simulink model "bergeron_100_segments"  (R2025b)
settings: Solver=FixedStepAuto  StartTime=0.0  StopTime=5/60  RelTol=1e-3
undefined symbols (not defined in the file): C0, C1, L0, L1, R0, R1, Ts
libraries: ee_lib_for_power_systems x200, ee_lib x5, nesl_utility x2, fl_lib x1
settings Model: Creator=gdudgeon  LastModifiedBy=gdudgeon

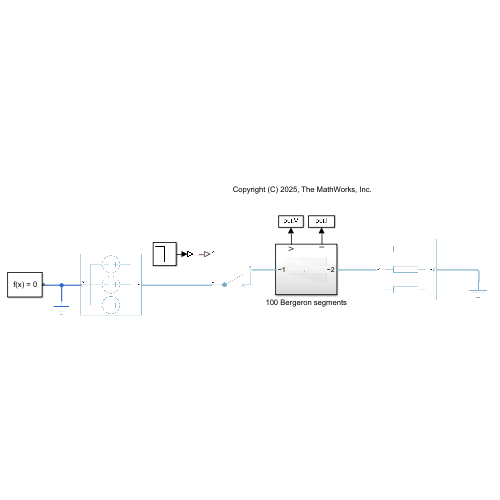
[thumbnail: Simulink's stored preview of the top-level diagram]
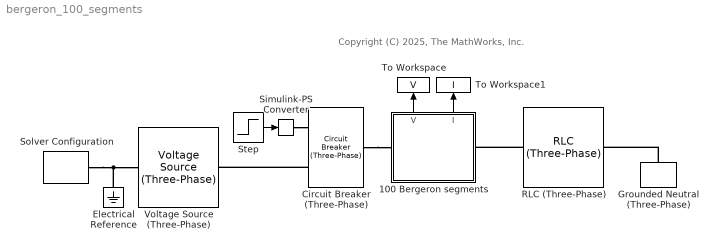
== system bergeron_100_segments ==
  note: Copyright (C) 2025, The MathWorks, Inc.
  100 Bergeron segments : Subsystem
      settings: PortSchema="{\"entries\":[{\"content\":{\"sides\":[{\"content\":{\"connectorIds\":[\"LConn1\"]},\"type\":\"ConnectorPlacement.EquallySpacedRectSide\",\"uuid\":\"b99b41a7-961a-494a-ac92-0b0e7e7066d5\"},{\"content\":{\"connectorIds\":[\"RConn1\"],\"side\":\"RIGHT\"},\"type\":\"ConnectorPlacement.EquallySpacedRectSide\",\"uuid\":\"a32a1a94-e4d8-4756-b184-838770a8045e\"},{\"content\":{\"connectorIds\":[\"Out1\",\"Out2\"],\"side\":\"TOP\"},\"type\":\"ConnectorPlacement.EquallySpacedRectSide\",\"uuid\":\"26c359be-d192-4d53-9097-18fe14f1011c\"},{\"content\":{\"side\":\"BOTTOM\"},\"type\":\"ConnectorPlacement.EquallySpacedRectSide\",\"uuid\":\"027abb80-d680-4e4d-9999-4a3aa56ae95f\"}]},\"type\":\"ConnectorPlacement.EquallySpacedConnector\",\"uuid\":\"03c9bddf-ebbb-4b3d-af53-face1d9ef075\"}],\"packageUris\":[\"http://schema.mathworks.com/mf0/Connector/R2020b\"],\"version\":\"1.0\"}"
  Circuit Breaker (Three-Phase) : ee_lib/Switches & Breakers/Circuit Breaker (Three-Phase)  R_closed=1e-6 Ohm  G_open=1e-6 1/Ohm  threshold=0.5 V  breaker_behavior=ee.enum.switches.breakerBehavior.zeroCrossingEnable
      settings: InternalSimscapePortConfiguration="{\"Bottom\":[],\"Left\":[{\"id\":\"vT\",\"label\":\"vT\",\"type\":\"input\"},{\"id\":\"N1\",\"label\":\"~1\",\"type\":\"foundation.electrical.three_phase\"}],\"Right\":[{\"id\":\"N2\",\"label\":\"~2\",\"type\":\"foundation.electrical.three_phase\"}],\"Top\":[]}"
  Electrical Reference : fl_lib/Electrical/Electrical Elements/Electrical Reference
  Grounded Neutral (Three-Phase) : ee_lib/Connectors & References/Grounded Neutral (Three-Phase)
  RLC (Three-Phase) : ee_lib/Passive/RLC Assemblies/RLC (Three-Phase)  port_option=ee.enum.threePhasePort.composite  component_structure=ee.enum.rlc.structure.SeriesRL  R=100 Ohm  L=1e-3 H  C=1e-6 F  R_parasitic=0 Ohm  G_parasitic=0 1/Ohm  IL_specify=off  IL_priority=High  IL=[0, 0, 0] A  IL_nominal_specify=off  IL_nominal_value=1  IL_nominal_unit=A  VC_specify=off  VC_priority=High  VC=[0, 0, 0] V  VC_nominal_specify=off  VC_nominal_value=1  VC_nominal_unit=V
      settings: InternalSimscapePortConfiguration="{\"Bottom\":[],\"Left\":[{\"id\":\"N1\",\"label\":\"~1\",\"type\":\"foundation.electrical.three_phase\"}],\"Right\":[{\"id\":\"N2\",\"label\":\"~2\",\"type\":\"foundation.electrical.three_phase\"}],\"Top\":[]}"
  Simulink-PS Converter : nesl_utility/Simulink-PS Converter  PhysicalDomain=network_engine_domain  SubClassName=ps_input  LeftPortType=input  RightPortType=output  PseudoPeriodic=off  Frequencies=[]  NoiseDistribution=none  NoiseParameters=[]  Unit=1  AffineConversion=off  FilteringAndDerivatives=provide  SimscapeFilterOrder=1  InputFilterTimeConstant=0.001  UdotUserProvided=0
  Solver Configuration : nesl_utility/Solver Configuration  PhysicalDomain=network_engine_domain  SubClassName=solver  LeftPortType=input  RightPortType=generic  Tones=[]  Harmonics=[]  SimulateNoise=off  Profile=off  UseLocalSampling=off  EnableSwitchedLinearOptims=on  FrequencyDomain=off  UseCCode=off  RelTol=0.001  AbsTol=0.001  MinStep=1e-09  ToWorkspace=off  RevertToSquareIcSolve=off  NumHomotopyIterations=100  PhasorMode=off  PhasorModeNumHarmonics=1  ConsistencySolver=NEWTON_XTOL_AFTER_FTOL  IndexReductionMethod=None  DoDC=off  ResidualTolerance=1e-09  ConsistencyTolSource=GLOBAL  ConsistencyAbsTol=0.001  ConsistencyRelTol=0.001  ConsistencyTolFactor=0.001  UseLocalSolver=on  LocalSolverChoice=NE_PARTITIONING_ADVANCER  ResolveIndetEquations=off  FunctionEvalNumThread=1  LocalSolverSampleTime=Ts  DoFixedCost=off  MaxNonlinIter=1  MaxModeIter=2  ComputeImpulses=off  ImpulseIterations=2  LinearAlgebra=auto  LinearAlgebraNumThread=0  EquationFormulation=NE_TIME_EF  DelaysMemoryBudget=1024  AutomaticFiltering=off  FilteringTimeConstant=0.001  PartitionStorageMethod=AS_NEEDED  PartitionMemoryBudget=1024  PartitionMethod=ROBUST  MultibodyUseLocalSolver=off  MultibodyLocalSolverChoice=ODE1  MultibodyLocalSolverSampleTime=0.001
  Step : Step  Time=0.1/60  Before=1  After=0  SampleTime=0
  To Workspace : ToWorkspace  VariableName=V  SaveFormat=Timeseries  SampleTime=Ts
  To Workspace1 : ToWorkspace  VariableName=I  SaveFormat=Timeseries  SampleTime=Ts
  Voltage Source (Three-Phase) : ee_lib/Sources/Voltage Source (Three-Phase)  vline_rms=100 V  shift=0 deg  freq=60 Hz  impedance_option=4  SShortCircuit=1e6 A*V  XR=15  R=0.01 Ohm  L=3.97e-4 H  harmonic_option=0  harmonic_orders=[5, 7, 11, 13]  harmonic_ratios=[.1, .1, .1, .1]  G_parasitic=0 1/Ohm  I_specify=off  I_priority=None  I=[0, 0, 0] A  I_nominal_specify=off  I_nominal_value=1  I_nominal_unit=A
  wires:
  Step/1 -> Simulink-PS Converter/1
  100 Bergeron segments/2(I) -> To Workspace1/1
  100 Bergeron segments/1(V) -> To Workspace/1
  connections:
  Electrical Reference/LConn1 -- Voltage Source (Three-Phase)/LConn1 -- Solver Configuration/RConn1
  Grounded Neutral (Three-Phase)/LConn1 -- RLC (Three-Phase)/RConn1
  Circuit Breaker (Three-Phase)/LConn2 -- Voltage Source (Three-Phase)/RConn1
  Circuit Breaker (Three-Phase)/RConn1 -- 100 Bergeron segments/LConn1
  RLC (Three-Phase)/LConn1 -- 100 Bergeron segments/RConn1
  Simulink-PS Converter/RConn1 -- Circuit Breaker (Three-Phase)/LConn1

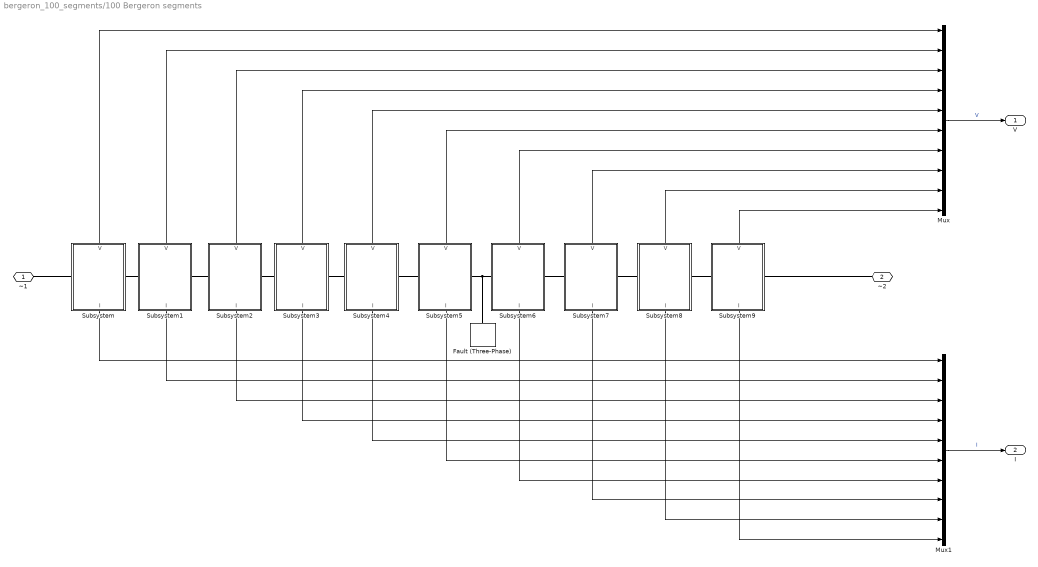
== system bergeron_100_segments/100 Bergeron segments ==
  Fault (Three-Phase) : ee_lib/Utilities/Fault (Three-Phase)  fault_type_option=11  R_pn_fault=1e-3 Ohm  R_ng_fault=1e-3 Ohm  exposemeasurement=ee.enum.exposemeasurement.hidden  enable_external_fault=ee.enum.external_fault.hidden  fault_threshold=0.5  fault_condition=1  fault_resettable=0  enable_temporal_fault=1  fault_start_time=2/60 s  fault_duration=0.001 s  G_parasitic=1e-6 1/Ohm
      settings: InternalSimscapePortConfiguration="{\"Bottom\":[],\"Left\":[{\"id\":\"N\",\"label\":\"~\",\"type\":\"foundation.electrical.three_phase\"}],\"Right\":[],\"Top\":[]}"
  Mux : Mux  Inputs=10
  Mux1 : Mux  Inputs=10
  Subsystem : Subsystem
      settings: PortSchema="{\"entries\":[{\"content\":{\"sides\":[{\"content\":{\"connectorIds\":[\"LConn1\"]},\"type\":\"ConnectorPlacement.EquallySpacedRectSide\",\"uuid\":\"be24dfa2-f72c-4790-92c4-42d34f360bf9\"},{\"content\":{\"connectorIds\":[\"RConn1\"],\"side\":\"RIGHT\"},\"type\":\"ConnectorPlacement.EquallySpacedRectSide\",\"uuid\":\"712463f8-85c9-4ba1-8bf5-09eaf7a29451\"},{\"content\":{\"connectorIds\":[\"Out2\"],\"side\":\"TOP\"},\"type\":\"ConnectorPlacement.EquallySpacedRectSide\",\"uuid\":\"03bd5c26-7b85-49ce-a0e2-a017bb2912ae\"},{\"content\":{\"connectorIds\":[\"Out1\"],\"side\":\"BOTTOM\"},\"type\":\"ConnectorPlacement.EquallySpacedRectSide\",\"uuid\":\"03e5b7e0-a176-4f73-96e3-dc5cabc5b21e\"}]},\"type\":\"ConnectorPlacement.EquallySpacedConnector\",\"uuid\":\"4458ec78-2ee4-4806-a1a7-ced2cc432a6e\"}],\"packageUris\":[\"http://schema.mathworks.com/mf0/Connector/R2020b\"],\"version\":\"1.0\"}"
  Subsystem1 : Subsystem
      settings: PortSchema="{\"entries\":[{\"content\":{\"sides\":[{\"content\":{\"connectorIds\":[\"LConn1\"]},\"type\":\"ConnectorPlacement.EquallySpacedRectSide\",\"uuid\":\"be24dfa2-f72c-4790-92c4-42d34f360bf9\"},{\"content\":{\"connectorIds\":[\"RConn1\"],\"side\":\"RIGHT\"},\"type\":\"ConnectorPlacement.EquallySpacedRectSide\",\"uuid\":\"712463f8-85c9-4ba1-8bf5-09eaf7a29451\"},{\"content\":{\"connectorIds\":[\"Out2\"],\"side\":\"TOP\"},\"type\":\"ConnectorPlacement.EquallySpacedRectSide\",\"uuid\":\"03bd5c26-7b85-49ce-a0e2-a017bb2912ae\"},{\"content\":{\"connectorIds\":[\"Out1\"],\"side\":\"BOTTOM\"},\"type\":\"ConnectorPlacement.EquallySpacedRectSide\",\"uuid\":\"03e5b7e0-a176-4f73-96e3-dc5cabc5b21e\"}]},\"type\":\"ConnectorPlacement.EquallySpacedConnector\",\"uuid\":\"4458ec78-2ee4-4806-a1a7-ced2cc432a6e\"}],\"packageUris\":[\"http://schema.mathworks.com/mf0/Connector/R2020b\"],\"version\":\"1.0\"}"
  Subsystem2 : Subsystem
      settings: PortSchema="{\"entries\":[{\"content\":{\"sides\":[{\"content\":{\"connectorIds\":[\"LConn1\"]},\"type\":\"ConnectorPlacement.EquallySpacedRectSide\",\"uuid\":\"be24dfa2-f72c-4790-92c4-42d34f360bf9\"},{\"content\":{\"connectorIds\":[\"RConn1\"],\"side\":\"RIGHT\"},\"type\":\"ConnectorPlacement.EquallySpacedRectSide\",\"uuid\":\"712463f8-85c9-4ba1-8bf5-09eaf7a29451\"},{\"content\":{\"connectorIds\":[\"Out2\"],\"side\":\"TOP\"},\"type\":\"ConnectorPlacement.EquallySpacedRectSide\",\"uuid\":\"03bd5c26-7b85-49ce-a0e2-a017bb2912ae\"},{\"content\":{\"connectorIds\":[\"Out1\"],\"side\":\"BOTTOM\"},\"type\":\"ConnectorPlacement.EquallySpacedRectSide\",\"uuid\":\"03e5b7e0-a176-4f73-96e3-dc5cabc5b21e\"}]},\"type\":\"ConnectorPlacement.EquallySpacedConnector\",\"uuid\":\"4458ec78-2ee4-4806-a1a7-ced2cc432a6e\"}],\"packageUris\":[\"http://schema.mathworks.com/mf0/Connector/R2020b\"],\"version\":\"1.0\"}"
  Subsystem3 : Subsystem
      settings: PortSchema="{\"entries\":[{\"content\":{\"sides\":[{\"content\":{\"connectorIds\":[\"LConn1\"]},\"type\":\"ConnectorPlacement.EquallySpacedRectSide\",\"uuid\":\"be24dfa2-f72c-4790-92c4-42d34f360bf9\"},{\"content\":{\"connectorIds\":[\"RConn1\"],\"side\":\"RIGHT\"},\"type\":\"ConnectorPlacement.EquallySpacedRectSide\",\"uuid\":\"712463f8-85c9-4ba1-8bf5-09eaf7a29451\"},{\"content\":{\"connectorIds\":[\"Out2\"],\"side\":\"TOP\"},\"type\":\"ConnectorPlacement.EquallySpacedRectSide\",\"uuid\":\"03bd5c26-7b85-49ce-a0e2-a017bb2912ae\"},{\"content\":{\"connectorIds\":[\"Out1\"],\"side\":\"BOTTOM\"},\"type\":\"ConnectorPlacement.EquallySpacedRectSide\",\"uuid\":\"03e5b7e0-a176-4f73-96e3-dc5cabc5b21e\"}]},\"type\":\"ConnectorPlacement.EquallySpacedConnector\",\"uuid\":\"4458ec78-2ee4-4806-a1a7-ced2cc432a6e\"}],\"packageUris\":[\"http://schema.mathworks.com/mf0/Connector/R2020b\"],\"version\":\"1.0\"}"
  Subsystem4 : Subsystem
      settings: PortSchema="{\"entries\":[{\"content\":{\"sides\":[{\"content\":{\"connectorIds\":[\"LConn1\"]},\"type\":\"ConnectorPlacement.EquallySpacedRectSide\",\"uuid\":\"be24dfa2-f72c-4790-92c4-42d34f360bf9\"},{\"content\":{\"connectorIds\":[\"RConn1\"],\"side\":\"RIGHT\"},\"type\":\"ConnectorPlacement.EquallySpacedRectSide\",\"uuid\":\"712463f8-85c9-4ba1-8bf5-09eaf7a29451\"},{\"content\":{\"connectorIds\":[\"Out2\"],\"side\":\"TOP\"},\"type\":\"ConnectorPlacement.EquallySpacedRectSide\",\"uuid\":\"03bd5c26-7b85-49ce-a0e2-a017bb2912ae\"},{\"content\":{\"connectorIds\":[\"Out1\"],\"side\":\"BOTTOM\"},\"type\":\"ConnectorPlacement.EquallySpacedRectSide\",\"uuid\":\"03e5b7e0-a176-4f73-96e3-dc5cabc5b21e\"}]},\"type\":\"ConnectorPlacement.EquallySpacedConnector\",\"uuid\":\"4458ec78-2ee4-4806-a1a7-ced2cc432a6e\"}],\"packageUris\":[\"http://schema.mathworks.com/mf0/Connector/R2020b\"],\"version\":\"1.0\"}"
  Subsystem5 : Subsystem
      settings: PortSchema="{\"entries\":[{\"content\":{\"sides\":[{\"content\":{\"connectorIds\":[\"LConn1\"]},\"type\":\"ConnectorPlacement.EquallySpacedRectSide\",\"uuid\":\"be24dfa2-f72c-4790-92c4-42d34f360bf9\"},{\"content\":{\"connectorIds\":[\"RConn1\"],\"side\":\"RIGHT\"},\"type\":\"ConnectorPlacement.EquallySpacedRectSide\",\"uuid\":\"712463f8-85c9-4ba1-8bf5-09eaf7a29451\"},{\"content\":{\"connectorIds\":[\"Out2\"],\"side\":\"TOP\"},\"type\":\"ConnectorPlacement.EquallySpacedRectSide\",\"uuid\":\"03bd5c26-7b85-49ce-a0e2-a017bb2912ae\"},{\"content\":{\"connectorIds\":[\"Out1\"],\"side\":\"BOTTOM\"},\"type\":\"ConnectorPlacement.EquallySpacedRectSide\",\"uuid\":\"03e5b7e0-a176-4f73-96e3-dc5cabc5b21e\"}]},\"type\":\"ConnectorPlacement.EquallySpacedConnector\",\"uuid\":\"4458ec78-2ee4-4806-a1a7-ced2cc432a6e\"}],\"packageUris\":[\"http://schema.mathworks.com/mf0/Connector/R2020b\"],\"version\":\"1.0\"}"
  Subsystem6 : Subsystem
      settings: PortSchema="{\"entries\":[{\"content\":{\"sides\":[{\"content\":{\"connectorIds\":[\"LConn1\"]},\"type\":\"ConnectorPlacement.EquallySpacedRectSide\",\"uuid\":\"be24dfa2-f72c-4790-92c4-42d34f360bf9\"},{\"content\":{\"connectorIds\":[\"RConn1\"],\"side\":\"RIGHT\"},\"type\":\"ConnectorPlacement.EquallySpacedRectSide\",\"uuid\":\"712463f8-85c9-4ba1-8bf5-09eaf7a29451\"},{\"content\":{\"connectorIds\":[\"Out2\"],\"side\":\"TOP\"},\"type\":\"ConnectorPlacement.EquallySpacedRectSide\",\"uuid\":\"03bd5c26-7b85-49ce-a0e2-a017bb2912ae\"},{\"content\":{\"connectorIds\":[\"Out1\"],\"side\":\"BOTTOM\"},\"type\":\"ConnectorPlacement.EquallySpacedRectSide\",\"uuid\":\"03e5b7e0-a176-4f73-96e3-dc5cabc5b21e\"}]},\"type\":\"ConnectorPlacement.EquallySpacedConnector\",\"uuid\":\"4458ec78-2ee4-4806-a1a7-ced2cc432a6e\"}],\"packageUris\":[\"http://schema.mathworks.com/mf0/Connector/R2020b\"],\"version\":\"1.0\"}"
  Subsystem7 : Subsystem
      settings: PortSchema="{\"entries\":[{\"content\":{\"sides\":[{\"content\":{\"connectorIds\":[\"LConn1\"]},\"type\":\"ConnectorPlacement.EquallySpacedRectSide\",\"uuid\":\"be24dfa2-f72c-4790-92c4-42d34f360bf9\"},{\"content\":{\"connectorIds\":[\"RConn1\"],\"side\":\"RIGHT\"},\"type\":\"ConnectorPlacement.EquallySpacedRectSide\",\"uuid\":\"712463f8-85c9-4ba1-8bf5-09eaf7a29451\"},{\"content\":{\"connectorIds\":[\"Out2\"],\"side\":\"TOP\"},\"type\":\"ConnectorPlacement.EquallySpacedRectSide\",\"uuid\":\"03bd5c26-7b85-49ce-a0e2-a017bb2912ae\"},{\"content\":{\"connectorIds\":[\"Out1\"],\"side\":\"BOTTOM\"},\"type\":\"ConnectorPlacement.EquallySpacedRectSide\",\"uuid\":\"03e5b7e0-a176-4f73-96e3-dc5cabc5b21e\"}]},\"type\":\"ConnectorPlacement.EquallySpacedConnector\",\"uuid\":\"4458ec78-2ee4-4806-a1a7-ced2cc432a6e\"}],\"packageUris\":[\"http://schema.mathworks.com/mf0/Connector/R2020b\"],\"version\":\"1.0\"}"
  Subsystem8 : Subsystem
      settings: PortSchema="{\"entries\":[{\"content\":{\"sides\":[{\"content\":{\"connectorIds\":[\"LConn1\"]},\"type\":\"ConnectorPlacement.EquallySpacedRectSide\",\"uuid\":\"be24dfa2-f72c-4790-92c4-42d34f360bf9\"},{\"content\":{\"connectorIds\":[\"RConn1\"],\"side\":\"RIGHT\"},\"type\":\"ConnectorPlacement.EquallySpacedRectSide\",\"uuid\":\"712463f8-85c9-4ba1-8bf5-09eaf7a29451\"},{\"content\":{\"connectorIds\":[\"Out2\"],\"side\":\"TOP\"},\"type\":\"ConnectorPlacement.EquallySpacedRectSide\",\"uuid\":\"03bd5c26-7b85-49ce-a0e2-a017bb2912ae\"},{\"content\":{\"connectorIds\":[\"Out1\"],\"side\":\"BOTTOM\"},\"type\":\"ConnectorPlacement.EquallySpacedRectSide\",\"uuid\":\"03e5b7e0-a176-4f73-96e3-dc5cabc5b21e\"}]},\"type\":\"ConnectorPlacement.EquallySpacedConnector\",\"uuid\":\"4458ec78-2ee4-4806-a1a7-ced2cc432a6e\"}],\"packageUris\":[\"http://schema.mathworks.com/mf0/Connector/R2020b\"],\"version\":\"1.0\"}"
  Subsystem9 : Subsystem
      settings: PortSchema="{\"entries\":[{\"content\":{\"sides\":[{\"content\":{\"connectorIds\":[\"LConn1\"]},\"type\":\"ConnectorPlacement.EquallySpacedRectSide\",\"uuid\":\"be24dfa2-f72c-4790-92c4-42d34f360bf9\"},{\"content\":{\"connectorIds\":[\"RConn1\"],\"side\":\"RIGHT\"},\"type\":\"ConnectorPlacement.EquallySpacedRectSide\",\"uuid\":\"712463f8-85c9-4ba1-8bf5-09eaf7a29451\"},{\"content\":{\"connectorIds\":[\"Out2\"],\"side\":\"TOP\"},\"type\":\"ConnectorPlacement.EquallySpacedRectSide\",\"uuid\":\"03bd5c26-7b85-49ce-a0e2-a017bb2912ae\"},{\"content\":{\"connectorIds\":[\"Out1\"],\"side\":\"BOTTOM\"},\"type\":\"ConnectorPlacement.EquallySpacedRectSide\",\"uuid\":\"03e5b7e0-a176-4f73-96e3-dc5cabc5b21e\"}]},\"type\":\"ConnectorPlacement.EquallySpacedConnector\",\"uuid\":\"4458ec78-2ee4-4806-a1a7-ced2cc432a6e\"}],\"packageUris\":[\"http://schema.mathworks.com/mf0/Connector/R2020b\"],\"version\":\"1.0\"}"
  ~1 : PMIOPort  Side=Left
  ~2 : PMIOPort  Port=2  Side=Right
  V : Outport
  I : Outport  Port=2
  wires:
  Subsystem9/1(I) -> Mux1/10
  Subsystem2/2(V) -> Mux/3
  Subsystem2/1(I) -> Mux1/3
  Subsystem1/2(V) -> Mux/2
  Subsystem6/2(V) -> Mux/7
  Subsystem5/1(I) -> Mux1/6
  Subsystem4/2(V) -> Mux/5
  Subsystem7/1(I) -> Mux1/8
  Subsystem7/2(V) -> Mux/8
  Subsystem5/2(V) -> Mux/6
  Subsystem/1(I) -> Mux1/1
  Subsystem6/1(I) -> Mux1/7
  Subsystem8/2(V) -> Mux/9
  Subsystem9/2(V) -> Mux/10
  Subsystem8/1(I) -> Mux1/9
  Subsystem3/1(I) -> Mux1/4
  Subsystem3/2(V) -> Mux/4
  Subsystem/2(V) -> Mux/1
  Subsystem4/1(I) -> Mux1/5
  Subsystem1/1(I) -> Mux1/2
  Mux1/1 -> I/1  "I"
  Mux/1 -> V/1  "V"
  connections:
  Subsystem3/RConn1 -- Subsystem4/LConn1
  Subsystem/LConn1 -- ~1/RConn1
  Subsystem9/RConn1 -- ~2/RConn1
  Subsystem7/LConn1 -- Subsystem6/RConn1
  Subsystem8/LConn1 -- Subsystem7/RConn1
  Fault (Three-Phase)/LConn1 -- Subsystem5/RConn1 -- Subsystem6/LConn1
  Subsystem5/LConn1 -- Subsystem4/RConn1
  Subsystem1/LConn1 -- Subsystem/RConn1
  Subsystem3/LConn1 -- Subsystem2/RConn1
  Subsystem2/LConn1 -- Subsystem1/RConn1
  Subsystem9/LConn1 -- Subsystem8/RConn1

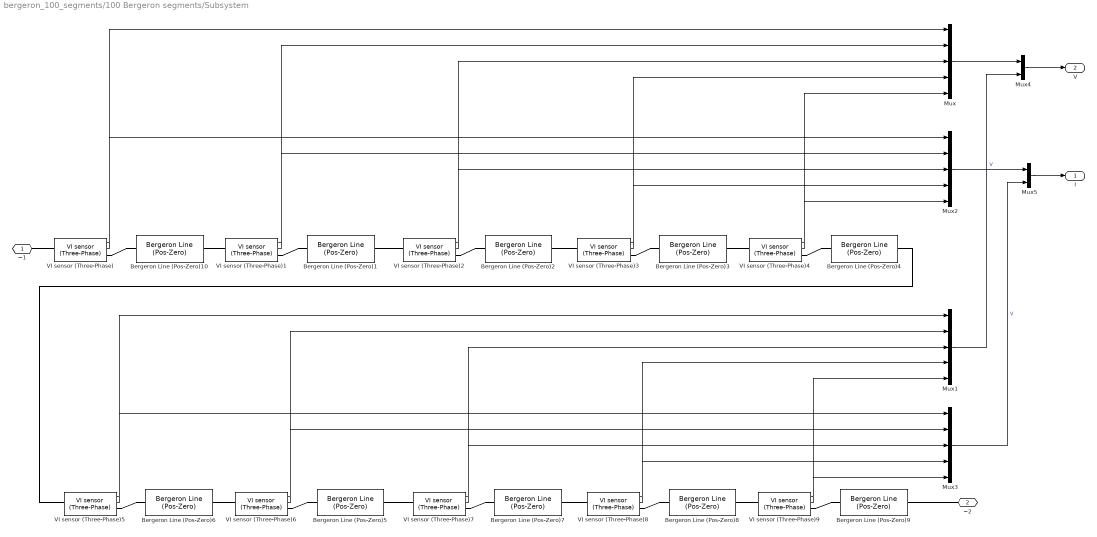
== system bergeron_100_segments/100 Bergeron segments/Subsystem ==
  Bergeron Line (Pos-Zero){1..10} (10 alike) : ee_lib_for_power_systems/Network Components/Bergeron Line (Pos-Zero)  length=length  R1_L1_C1=[R1 L1 C1]  R0_L0_C0=[R0 L0 C0]  Ts=Ts
      settings: SourceProductName=Support Library for Power Systems
  Mux{,1..3} (4 alike) : Mux  Inputs=5
  Mux4 : Mux  Inputs=2
  Mux5 : Mux  Inputs=2
  VI sensor (Three-Phase){,1..9} (10 alike) : ee_lib_for_power_systems/Sense and Measure/VI sensor (Three-Phase)  volt_meas=Phase-to-Ground (Phase Voltage)  meas_units=SI  Vnom=24e3  Pnom=100e6
      settings: SourceProductName=Support Library for Power Systems
  ~1 : PMIOPort  Side=Left
  ~2 : PMIOPort  Port=2  Side=Right
  I : Outport
  V : Outport  Port=2
  wires:
  VI sensor (Three-Phase)/1 -> Mux/1
  VI sensor (Three-Phase)1/1 -> Mux/2
  VI sensor (Three-Phase)2/1 -> Mux/3
  VI sensor (Three-Phase)3/1 -> Mux/4
  VI sensor (Three-Phase)4/1 -> Mux/5
  VI sensor (Three-Phase)/2 -> Mux2/1
  VI sensor (Three-Phase)1/2 -> Mux2/2
  VI sensor (Three-Phase)2/2 -> Mux2/3
  VI sensor (Three-Phase)3/2 -> Mux2/4
  VI sensor (Three-Phase)4/2 -> Mux2/5
  VI sensor (Three-Phase)5/1 -> Mux1/1
  VI sensor (Three-Phase)6/1 -> Mux1/2
  VI sensor (Three-Phase)7/1 -> Mux1/3
  VI sensor (Three-Phase)8/1 -> Mux1/4
  VI sensor (Three-Phase)9/1 -> Mux1/5
  VI sensor (Three-Phase)5/2 -> Mux3/1
  VI sensor (Three-Phase)6/2 -> Mux3/2
  VI sensor (Three-Phase)7/2 -> Mux3/3
  VI sensor (Three-Phase)8/2 -> Mux3/4
  VI sensor (Three-Phase)9/2 -> Mux3/5
  Mux/1 -> Mux4/1
  Mux1/1 -> Mux4/2
  Mux4/1 -> V/1
  Mux2/1 -> Mux5/1  "V"
  Mux3/1 -> Mux5/2  "V"
  Mux5/1 -> I/1
  connections:
  Bergeron Line (Pos-Zero)10/LConn1 -- VI sensor (Three-Phase)/RConn1
  VI sensor (Three-Phase)/LConn1 -- ~1/RConn1
  VI sensor (Three-Phase)1/LConn1 -- Bergeron Line (Pos-Zero)10/RConn1
  ~2/RConn1 -- Bergeron Line (Pos-Zero)9/RConn1
  Bergeron Line (Pos-Zero)1/LConn1 -- VI sensor (Three-Phase)1/RConn1
  Bergeron Line (Pos-Zero)2/LConn1 -- VI sensor (Three-Phase)2/RConn1
  VI sensor (Three-Phase)2/LConn1 -- Bergeron Line (Pos-Zero)1/RConn1
  Bergeron Line (Pos-Zero)3/LConn1 -- VI sensor (Three-Phase)3/RConn1
  VI sensor (Three-Phase)3/LConn1 -- Bergeron Line (Pos-Zero)2/RConn1
  Bergeron Line (Pos-Zero)4/LConn1 -- VI sensor (Three-Phase)4/RConn1
  Bergeron Line (Pos-Zero)3/RConn1 -- VI sensor (Three-Phase)4/LConn1
  Bergeron Line (Pos-Zero)8/RConn1 -- VI sensor (Three-Phase)9/LConn1
  Bergeron Line (Pos-Zero)9/LConn1 -- VI sensor (Three-Phase)9/RConn1
  VI sensor (Three-Phase)7/LConn1 -- Bergeron Line (Pos-Zero)5/RConn1
  Bergeron Line (Pos-Zero)8/LConn1 -- VI sensor (Three-Phase)8/RConn1
  Bergeron Line (Pos-Zero)7/LConn1 -- VI sensor (Three-Phase)7/RConn1
  Bergeron Line (Pos-Zero)5/LConn1 -- VI sensor (Three-Phase)6/RConn1
  VI sensor (Three-Phase)6/LConn1 -- Bergeron Line (Pos-Zero)6/RConn1
  Bergeron Line (Pos-Zero)6/LConn1 -- VI sensor (Three-Phase)5/RConn1
  VI sensor (Three-Phase)8/LConn1 -- Bergeron Line (Pos-Zero)7/RConn1
  VI sensor (Three-Phase)5/LConn1 -- Bergeron Line (Pos-Zero)4/RConn1

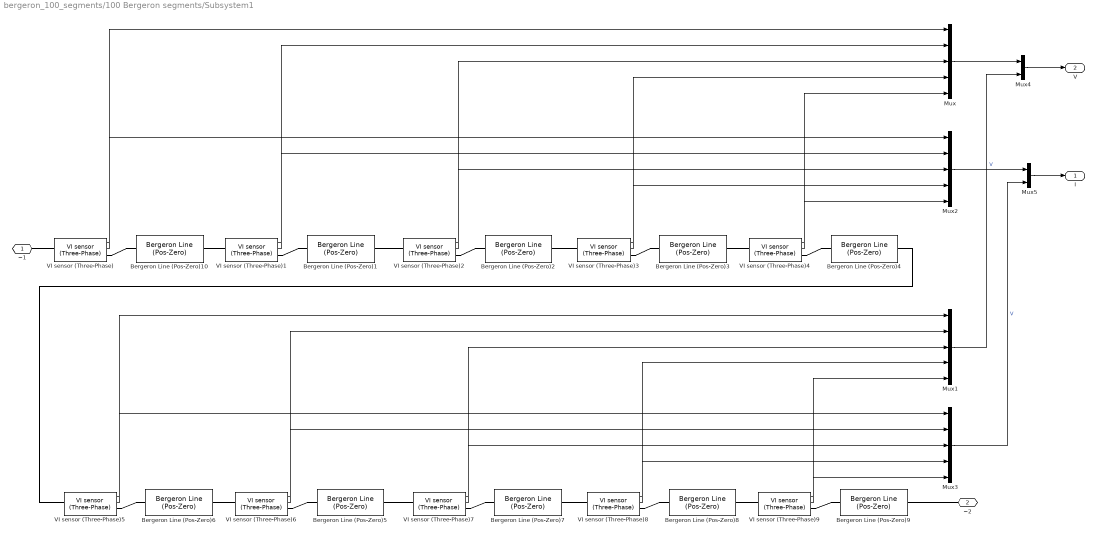
== system bergeron_100_segments/100 Bergeron segments/Subsystem1 ==
  Bergeron Line (Pos-Zero){1..10} (10 alike) : ee_lib_for_power_systems/Network Components/Bergeron Line (Pos-Zero)  length=length  R1_L1_C1=[R1 L1 C1]  R0_L0_C0=[R0 L0 C0]  Ts=Ts
      settings: SourceProductName=Support Library for Power Systems
  Mux{,1..3} (4 alike) : Mux  Inputs=5
  Mux4 : Mux  Inputs=2
  Mux5 : Mux  Inputs=2
  VI sensor (Three-Phase){,1..9} (10 alike) : ee_lib_for_power_systems/Sense and Measure/VI sensor (Three-Phase)  volt_meas=Phase-to-Ground (Phase Voltage)  meas_units=SI  Vnom=24e3  Pnom=100e6
      settings: SourceProductName=Support Library for Power Systems
  ~1 : PMIOPort  Side=Left
  ~2 : PMIOPort  Port=2  Side=Right
  I : Outport
  V : Outport  Port=2
  wires:
  Mux5/1 -> I/1
  Mux3/1 -> Mux5/2  "V"
  Mux2/1 -> Mux5/1  "V"
  Mux4/1 -> V/1
  Mux1/1 -> Mux4/2
  Mux/1 -> Mux4/1
  VI sensor (Three-Phase)9/2 -> Mux3/5
  VI sensor (Three-Phase)8/2 -> Mux3/4
  VI sensor (Three-Phase)7/2 -> Mux3/3
  VI sensor (Three-Phase)6/2 -> Mux3/2
  VI sensor (Three-Phase)5/2 -> Mux3/1
  VI sensor (Three-Phase)9/1 -> Mux1/5
  VI sensor (Three-Phase)8/1 -> Mux1/4
  VI sensor (Three-Phase)7/1 -> Mux1/3
  VI sensor (Three-Phase)6/1 -> Mux1/2
  VI sensor (Three-Phase)5/1 -> Mux1/1
  VI sensor (Three-Phase)4/2 -> Mux2/5
  VI sensor (Three-Phase)3/2 -> Mux2/4
  VI sensor (Three-Phase)2/2 -> Mux2/3
  VI sensor (Three-Phase)1/2 -> Mux2/2
  VI sensor (Three-Phase)/2 -> Mux2/1
  VI sensor (Three-Phase)4/1 -> Mux/5
  VI sensor (Three-Phase)3/1 -> Mux/4
  VI sensor (Three-Phase)2/1 -> Mux/3
  VI sensor (Three-Phase)1/1 -> Mux/2
  VI sensor (Three-Phase)/1 -> Mux/1
  connections:
  VI sensor (Three-Phase)5/LConn1 -- Bergeron Line (Pos-Zero)4/RConn1
  VI sensor (Three-Phase)8/LConn1 -- Bergeron Line (Pos-Zero)7/RConn1
  Bergeron Line (Pos-Zero)6/LConn1 -- VI sensor (Three-Phase)5/RConn1
  VI sensor (Three-Phase)6/LConn1 -- Bergeron Line (Pos-Zero)6/RConn1
  Bergeron Line (Pos-Zero)5/LConn1 -- VI sensor (Three-Phase)6/RConn1
  Bergeron Line (Pos-Zero)7/LConn1 -- VI sensor (Three-Phase)7/RConn1
  Bergeron Line (Pos-Zero)8/LConn1 -- VI sensor (Three-Phase)8/RConn1
  VI sensor (Three-Phase)7/LConn1 -- Bergeron Line (Pos-Zero)5/RConn1
  Bergeron Line (Pos-Zero)9/LConn1 -- VI sensor (Three-Phase)9/RConn1
  Bergeron Line (Pos-Zero)8/RConn1 -- VI sensor (Three-Phase)9/LConn1
  Bergeron Line (Pos-Zero)3/RConn1 -- VI sensor (Three-Phase)4/LConn1
  Bergeron Line (Pos-Zero)4/LConn1 -- VI sensor (Three-Phase)4/RConn1
  VI sensor (Three-Phase)3/LConn1 -- Bergeron Line (Pos-Zero)2/RConn1
  Bergeron Line (Pos-Zero)3/LConn1 -- VI sensor (Three-Phase)3/RConn1
  VI sensor (Three-Phase)2/LConn1 -- Bergeron Line (Pos-Zero)1/RConn1
  Bergeron Line (Pos-Zero)2/LConn1 -- VI sensor (Three-Phase)2/RConn1
  Bergeron Line (Pos-Zero)1/LConn1 -- VI sensor (Three-Phase)1/RConn1
  ~2/RConn1 -- Bergeron Line (Pos-Zero)9/RConn1
  VI sensor (Three-Phase)1/LConn1 -- Bergeron Line (Pos-Zero)10/RConn1
  VI sensor (Three-Phase)/LConn1 -- ~1/RConn1
  Bergeron Line (Pos-Zero)10/LConn1 -- VI sensor (Three-Phase)/RConn1

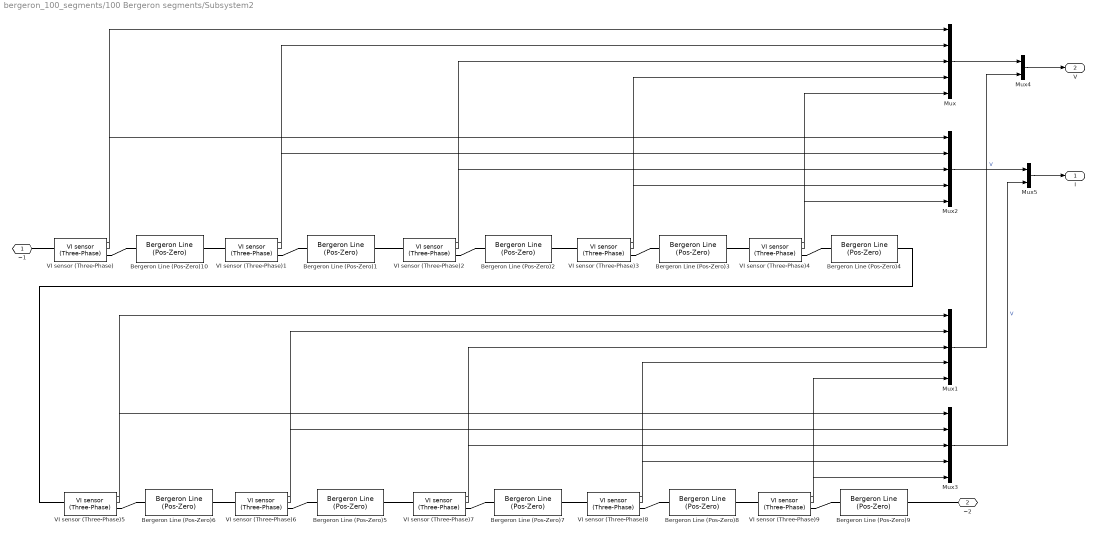
== system bergeron_100_segments/100 Bergeron segments/Subsystem2 ==
  Bergeron Line (Pos-Zero){1..10} (10 alike) : ee_lib_for_power_systems/Network Components/Bergeron Line (Pos-Zero)  length=length  R1_L1_C1=[R1 L1 C1]  R0_L0_C0=[R0 L0 C0]  Ts=Ts
      settings: SourceProductName=Support Library for Power Systems
  Mux{,1..3} (4 alike) : Mux  Inputs=5
  Mux4 : Mux  Inputs=2
  Mux5 : Mux  Inputs=2
  VI sensor (Three-Phase){,1..9} (10 alike) : ee_lib_for_power_systems/Sense and Measure/VI sensor (Three-Phase)  volt_meas=Phase-to-Ground (Phase Voltage)  meas_units=SI  Vnom=24e3  Pnom=100e6
      settings: SourceProductName=Support Library for Power Systems
  ~1 : PMIOPort  Side=Left
  ~2 : PMIOPort  Port=2  Side=Right
  I : Outport
  V : Outport  Port=2
  wires:
  VI sensor (Three-Phase)/1 -> Mux/1
  VI sensor (Three-Phase)1/1 -> Mux/2
  VI sensor (Three-Phase)2/1 -> Mux/3
  VI sensor (Three-Phase)3/1 -> Mux/4
  VI sensor (Three-Phase)4/1 -> Mux/5
  VI sensor (Three-Phase)/2 -> Mux2/1
  VI sensor (Three-Phase)1/2 -> Mux2/2
  VI sensor (Three-Phase)2/2 -> Mux2/3
  VI sensor (Three-Phase)3/2 -> Mux2/4
  VI sensor (Three-Phase)4/2 -> Mux2/5
  VI sensor (Three-Phase)5/1 -> Mux1/1
  VI sensor (Three-Phase)6/1 -> Mux1/2
  VI sensor (Three-Phase)7/1 -> Mux1/3
  VI sensor (Three-Phase)8/1 -> Mux1/4
  VI sensor (Three-Phase)9/1 -> Mux1/5
  VI sensor (Three-Phase)5/2 -> Mux3/1
  VI sensor (Three-Phase)6/2 -> Mux3/2
  VI sensor (Three-Phase)7/2 -> Mux3/3
  VI sensor (Three-Phase)8/2 -> Mux3/4
  VI sensor (Three-Phase)9/2 -> Mux3/5
  Mux/1 -> Mux4/1
  Mux1/1 -> Mux4/2
  Mux4/1 -> V/1
  Mux2/1 -> Mux5/1  "V"
  Mux3/1 -> Mux5/2  "V"
  Mux5/1 -> I/1
  connections:
  Bergeron Line (Pos-Zero)10/LConn1 -- VI sensor (Three-Phase)/RConn1
  VI sensor (Three-Phase)/LConn1 -- ~1/RConn1
  VI sensor (Three-Phase)1/LConn1 -- Bergeron Line (Pos-Zero)10/RConn1
  ~2/RConn1 -- Bergeron Line (Pos-Zero)9/RConn1
  Bergeron Line (Pos-Zero)1/LConn1 -- VI sensor (Three-Phase)1/RConn1
  Bergeron Line (Pos-Zero)2/LConn1 -- VI sensor (Three-Phase)2/RConn1
  VI sensor (Three-Phase)2/LConn1 -- Bergeron Line (Pos-Zero)1/RConn1
  Bergeron Line (Pos-Zero)3/LConn1 -- VI sensor (Three-Phase)3/RConn1
  VI sensor (Three-Phase)3/LConn1 -- Bergeron Line (Pos-Zero)2/RConn1
  Bergeron Line (Pos-Zero)4/LConn1 -- VI sensor (Three-Phase)4/RConn1
  Bergeron Line (Pos-Zero)3/RConn1 -- VI sensor (Three-Phase)4/LConn1
  Bergeron Line (Pos-Zero)8/RConn1 -- VI sensor (Three-Phase)9/LConn1
  Bergeron Line (Pos-Zero)9/LConn1 -- VI sensor (Three-Phase)9/RConn1
  VI sensor (Three-Phase)7/LConn1 -- Bergeron Line (Pos-Zero)5/RConn1
  Bergeron Line (Pos-Zero)8/LConn1 -- VI sensor (Three-Phase)8/RConn1
  Bergeron Line (Pos-Zero)7/LConn1 -- VI sensor (Three-Phase)7/RConn1
  Bergeron Line (Pos-Zero)5/LConn1 -- VI sensor (Three-Phase)6/RConn1
  VI sensor (Three-Phase)6/LConn1 -- Bergeron Line (Pos-Zero)6/RConn1
  Bergeron Line (Pos-Zero)6/LConn1 -- VI sensor (Three-Phase)5/RConn1
  VI sensor (Three-Phase)8/LConn1 -- Bergeron Line (Pos-Zero)7/RConn1
  VI sensor (Three-Phase)5/LConn1 -- Bergeron Line (Pos-Zero)4/RConn1

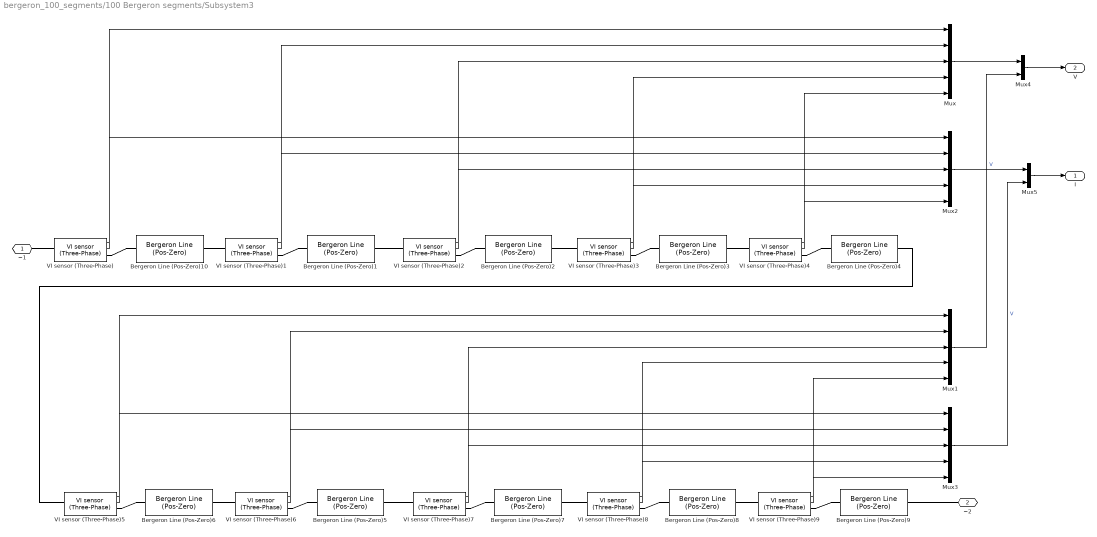
== system bergeron_100_segments/100 Bergeron segments/Subsystem3 ==
  Bergeron Line (Pos-Zero){1..10} (10 alike) : ee_lib_for_power_systems/Network Components/Bergeron Line (Pos-Zero)  length=length  R1_L1_C1=[R1 L1 C1]  R0_L0_C0=[R0 L0 C0]  Ts=Ts
      settings: SourceProductName=Support Library for Power Systems
  Mux{,1..3} (4 alike) : Mux  Inputs=5
  Mux4 : Mux  Inputs=2
  Mux5 : Mux  Inputs=2
  VI sensor (Three-Phase){,1..9} (10 alike) : ee_lib_for_power_systems/Sense and Measure/VI sensor (Three-Phase)  volt_meas=Phase-to-Ground (Phase Voltage)  meas_units=SI  Vnom=24e3  Pnom=100e6
      settings: SourceProductName=Support Library for Power Systems
  ~1 : PMIOPort  Side=Left
  ~2 : PMIOPort  Port=2  Side=Right
  I : Outport
  V : Outport  Port=2
  wires:
  Mux5/1 -> I/1
  Mux3/1 -> Mux5/2  "V"
  Mux2/1 -> Mux5/1  "V"
  Mux4/1 -> V/1
  Mux1/1 -> Mux4/2
  Mux/1 -> Mux4/1
  VI sensor (Three-Phase)9/2 -> Mux3/5
  VI sensor (Three-Phase)8/2 -> Mux3/4
  VI sensor (Three-Phase)7/2 -> Mux3/3
  VI sensor (Three-Phase)6/2 -> Mux3/2
  VI sensor (Three-Phase)5/2 -> Mux3/1
  VI sensor (Three-Phase)9/1 -> Mux1/5
  VI sensor (Three-Phase)8/1 -> Mux1/4
  VI sensor (Three-Phase)7/1 -> Mux1/3
  VI sensor (Three-Phase)6/1 -> Mux1/2
  VI sensor (Three-Phase)5/1 -> Mux1/1
  VI sensor (Three-Phase)4/2 -> Mux2/5
  VI sensor (Three-Phase)3/2 -> Mux2/4
  VI sensor (Three-Phase)2/2 -> Mux2/3
  VI sensor (Three-Phase)1/2 -> Mux2/2
  VI sensor (Three-Phase)/2 -> Mux2/1
  VI sensor (Three-Phase)4/1 -> Mux/5
  VI sensor (Three-Phase)3/1 -> Mux/4
  VI sensor (Three-Phase)2/1 -> Mux/3
  VI sensor (Three-Phase)1/1 -> Mux/2
  VI sensor (Three-Phase)/1 -> Mux/1
  connections:
  VI sensor (Three-Phase)5/LConn1 -- Bergeron Line (Pos-Zero)4/RConn1
  VI sensor (Three-Phase)8/LConn1 -- Bergeron Line (Pos-Zero)7/RConn1
  Bergeron Line (Pos-Zero)6/LConn1 -- VI sensor (Three-Phase)5/RConn1
  VI sensor (Three-Phase)6/LConn1 -- Bergeron Line (Pos-Zero)6/RConn1
  Bergeron Line (Pos-Zero)5/LConn1 -- VI sensor (Three-Phase)6/RConn1
  Bergeron Line (Pos-Zero)7/LConn1 -- VI sensor (Three-Phase)7/RConn1
  Bergeron Line (Pos-Zero)8/LConn1 -- VI sensor (Three-Phase)8/RConn1
  VI sensor (Three-Phase)7/LConn1 -- Bergeron Line (Pos-Zero)5/RConn1
  Bergeron Line (Pos-Zero)9/LConn1 -- VI sensor (Three-Phase)9/RConn1
  Bergeron Line (Pos-Zero)8/RConn1 -- VI sensor (Three-Phase)9/LConn1
  Bergeron Line (Pos-Zero)3/RConn1 -- VI sensor (Three-Phase)4/LConn1
  Bergeron Line (Pos-Zero)4/LConn1 -- VI sensor (Three-Phase)4/RConn1
  VI sensor (Three-Phase)3/LConn1 -- Bergeron Line (Pos-Zero)2/RConn1
  Bergeron Line (Pos-Zero)3/LConn1 -- VI sensor (Three-Phase)3/RConn1
  VI sensor (Three-Phase)2/LConn1 -- Bergeron Line (Pos-Zero)1/RConn1
  Bergeron Line (Pos-Zero)2/LConn1 -- VI sensor (Three-Phase)2/RConn1
  Bergeron Line (Pos-Zero)1/LConn1 -- VI sensor (Three-Phase)1/RConn1
  ~2/RConn1 -- Bergeron Line (Pos-Zero)9/RConn1
  VI sensor (Three-Phase)1/LConn1 -- Bergeron Line (Pos-Zero)10/RConn1
  VI sensor (Three-Phase)/LConn1 -- ~1/RConn1
  Bergeron Line (Pos-Zero)10/LConn1 -- VI sensor (Three-Phase)/RConn1

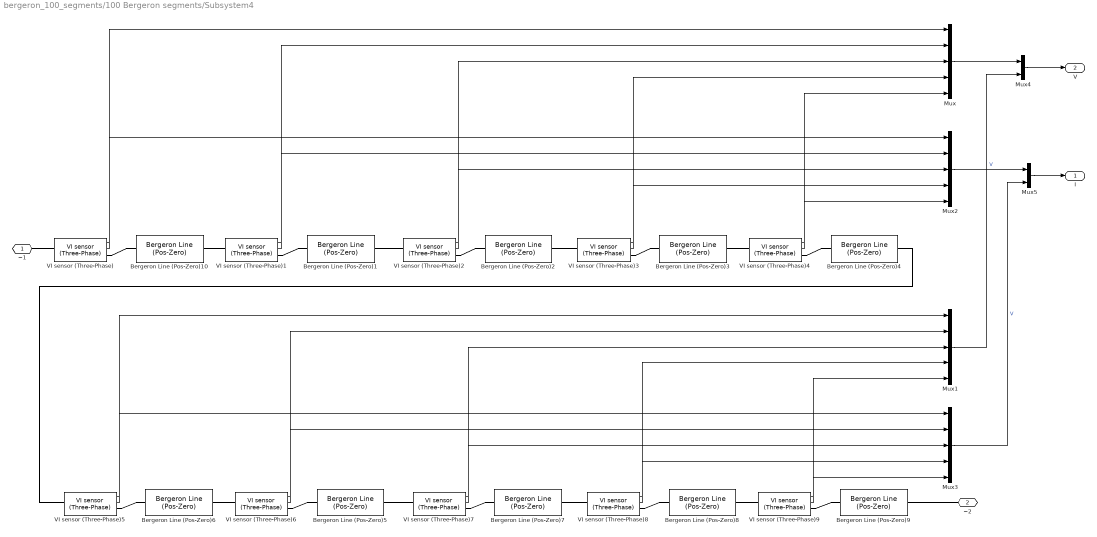
== system bergeron_100_segments/100 Bergeron segments/Subsystem4 ==
  Bergeron Line (Pos-Zero){1..10} (10 alike) : ee_lib_for_power_systems/Network Components/Bergeron Line (Pos-Zero)  length=length  R1_L1_C1=[R1 L1 C1]  R0_L0_C0=[R0 L0 C0]  Ts=Ts
      settings: SourceProductName=Support Library for Power Systems
  Mux{,1..3} (4 alike) : Mux  Inputs=5
  Mux4 : Mux  Inputs=2
  Mux5 : Mux  Inputs=2
  VI sensor (Three-Phase){,1..9} (10 alike) : ee_lib_for_power_systems/Sense and Measure/VI sensor (Three-Phase)  volt_meas=Phase-to-Ground (Phase Voltage)  meas_units=SI  Vnom=24e3  Pnom=100e6
      settings: SourceProductName=Support Library for Power Systems
  ~1 : PMIOPort  Side=Left
  ~2 : PMIOPort  Port=2  Side=Right
  I : Outport
  V : Outport  Port=2
  wires:
  VI sensor (Three-Phase)/1 -> Mux/1
  VI sensor (Three-Phase)1/1 -> Mux/2
  VI sensor (Three-Phase)2/1 -> Mux/3
  VI sensor (Three-Phase)3/1 -> Mux/4
  VI sensor (Three-Phase)4/1 -> Mux/5
  VI sensor (Three-Phase)/2 -> Mux2/1
  VI sensor (Three-Phase)1/2 -> Mux2/2
  VI sensor (Three-Phase)2/2 -> Mux2/3
  VI sensor (Three-Phase)3/2 -> Mux2/4
  VI sensor (Three-Phase)4/2 -> Mux2/5
  VI sensor (Three-Phase)5/1 -> Mux1/1
  VI sensor (Three-Phase)6/1 -> Mux1/2
  VI sensor (Three-Phase)7/1 -> Mux1/3
  VI sensor (Three-Phase)8/1 -> Mux1/4
  VI sensor (Three-Phase)9/1 -> Mux1/5
  VI sensor (Three-Phase)5/2 -> Mux3/1
  VI sensor (Three-Phase)6/2 -> Mux3/2
  VI sensor (Three-Phase)7/2 -> Mux3/3
  VI sensor (Three-Phase)8/2 -> Mux3/4
  VI sensor (Three-Phase)9/2 -> Mux3/5
  Mux/1 -> Mux4/1
  Mux1/1 -> Mux4/2
  Mux4/1 -> V/1
  Mux2/1 -> Mux5/1  "V"
  Mux3/1 -> Mux5/2  "V"
  Mux5/1 -> I/1
  connections:
  Bergeron Line (Pos-Zero)10/LConn1 -- VI sensor (Three-Phase)/RConn1
  VI sensor (Three-Phase)/LConn1 -- ~1/RConn1
  VI sensor (Three-Phase)1/LConn1 -- Bergeron Line (Pos-Zero)10/RConn1
  ~2/RConn1 -- Bergeron Line (Pos-Zero)9/RConn1
  Bergeron Line (Pos-Zero)1/LConn1 -- VI sensor (Three-Phase)1/RConn1
  Bergeron Line (Pos-Zero)2/LConn1 -- VI sensor (Three-Phase)2/RConn1
  VI sensor (Three-Phase)2/LConn1 -- Bergeron Line (Pos-Zero)1/RConn1
  Bergeron Line (Pos-Zero)3/LConn1 -- VI sensor (Three-Phase)3/RConn1
  VI sensor (Three-Phase)3/LConn1 -- Bergeron Line (Pos-Zero)2/RConn1
  Bergeron Line (Pos-Zero)4/LConn1 -- VI sensor (Three-Phase)4/RConn1
  Bergeron Line (Pos-Zero)3/RConn1 -- VI sensor (Three-Phase)4/LConn1
  Bergeron Line (Pos-Zero)8/RConn1 -- VI sensor (Three-Phase)9/LConn1
  Bergeron Line (Pos-Zero)9/LConn1 -- VI sensor (Three-Phase)9/RConn1
  VI sensor (Three-Phase)7/LConn1 -- Bergeron Line (Pos-Zero)5/RConn1
  Bergeron Line (Pos-Zero)8/LConn1 -- VI sensor (Three-Phase)8/RConn1
  Bergeron Line (Pos-Zero)7/LConn1 -- VI sensor (Three-Phase)7/RConn1
  Bergeron Line (Pos-Zero)5/LConn1 -- VI sensor (Three-Phase)6/RConn1
  VI sensor (Three-Phase)6/LConn1 -- Bergeron Line (Pos-Zero)6/RConn1
  Bergeron Line (Pos-Zero)6/LConn1 -- VI sensor (Three-Phase)5/RConn1
  VI sensor (Three-Phase)8/LConn1 -- Bergeron Line (Pos-Zero)7/RConn1
  VI sensor (Three-Phase)5/LConn1 -- Bergeron Line (Pos-Zero)4/RConn1

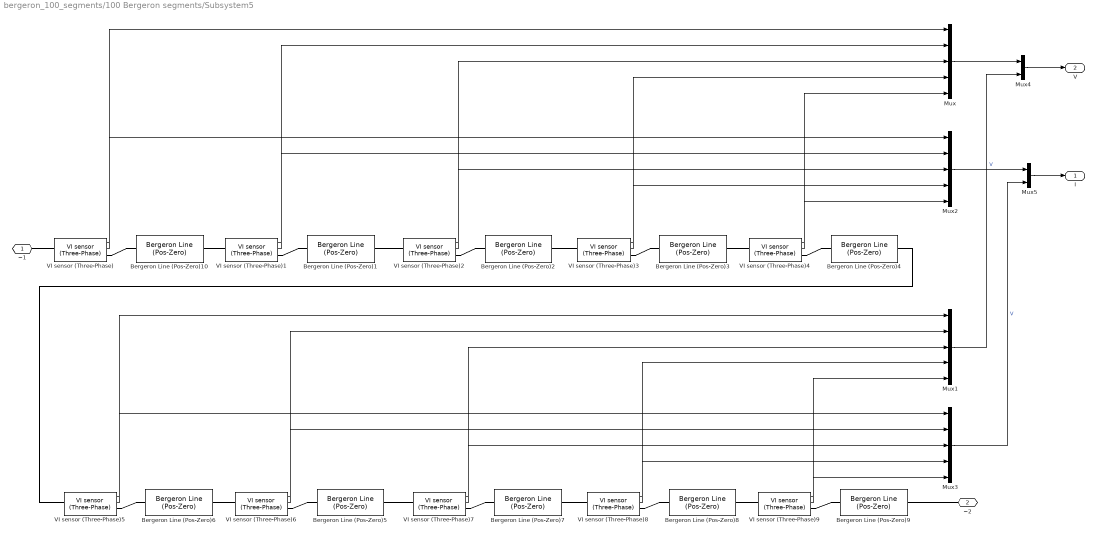
== system bergeron_100_segments/100 Bergeron segments/Subsystem5 ==
  Bergeron Line (Pos-Zero){1..10} (10 alike) : ee_lib_for_power_systems/Network Components/Bergeron Line (Pos-Zero)  length=length  R1_L1_C1=[R1 L1 C1]  R0_L0_C0=[R0 L0 C0]  Ts=Ts
      settings: SourceProductName=Support Library for Power Systems
  Mux{,1..3} (4 alike) : Mux  Inputs=5
  Mux4 : Mux  Inputs=2
  Mux5 : Mux  Inputs=2
  VI sensor (Three-Phase){,1..9} (10 alike) : ee_lib_for_power_systems/Sense and Measure/VI sensor (Three-Phase)  volt_meas=Phase-to-Ground (Phase Voltage)  meas_units=SI  Vnom=24e3  Pnom=100e6
      settings: SourceProductName=Support Library for Power Systems
  ~1 : PMIOPort  Side=Left
  ~2 : PMIOPort  Port=2  Side=Right
  I : Outport
  V : Outport  Port=2
  wires:
  Mux5/1 -> I/1
  Mux3/1 -> Mux5/2  "V"
  Mux2/1 -> Mux5/1  "V"
  Mux4/1 -> V/1
  Mux1/1 -> Mux4/2
  Mux/1 -> Mux4/1
  VI sensor (Three-Phase)9/2 -> Mux3/5
  VI sensor (Three-Phase)8/2 -> Mux3/4
  VI sensor (Three-Phase)7/2 -> Mux3/3
  VI sensor (Three-Phase)6/2 -> Mux3/2
  VI sensor (Three-Phase)5/2 -> Mux3/1
  VI sensor (Three-Phase)9/1 -> Mux1/5
  VI sensor (Three-Phase)8/1 -> Mux1/4
  VI sensor (Three-Phase)7/1 -> Mux1/3
  VI sensor (Three-Phase)6/1 -> Mux1/2
  VI sensor (Three-Phase)5/1 -> Mux1/1
  VI sensor (Three-Phase)4/2 -> Mux2/5
  VI sensor (Three-Phase)3/2 -> Mux2/4
  VI sensor (Three-Phase)2/2 -> Mux2/3
  VI sensor (Three-Phase)1/2 -> Mux2/2
  VI sensor (Three-Phase)/2 -> Mux2/1
  VI sensor (Three-Phase)4/1 -> Mux/5
  VI sensor (Three-Phase)3/1 -> Mux/4
  VI sensor (Three-Phase)2/1 -> Mux/3
  VI sensor (Three-Phase)1/1 -> Mux/2
  VI sensor (Three-Phase)/1 -> Mux/1
  connections:
  VI sensor (Three-Phase)5/LConn1 -- Bergeron Line (Pos-Zero)4/RConn1
  VI sensor (Three-Phase)8/LConn1 -- Bergeron Line (Pos-Zero)7/RConn1
  Bergeron Line (Pos-Zero)6/LConn1 -- VI sensor (Three-Phase)5/RConn1
  VI sensor (Three-Phase)6/LConn1 -- Bergeron Line (Pos-Zero)6/RConn1
  Bergeron Line (Pos-Zero)5/LConn1 -- VI sensor (Three-Phase)6/RConn1
  Bergeron Line (Pos-Zero)7/LConn1 -- VI sensor (Three-Phase)7/RConn1
  Bergeron Line (Pos-Zero)8/LConn1 -- VI sensor (Three-Phase)8/RConn1
  VI sensor (Three-Phase)7/LConn1 -- Bergeron Line (Pos-Zero)5/RConn1
  Bergeron Line (Pos-Zero)9/LConn1 -- VI sensor (Three-Phase)9/RConn1
  Bergeron Line (Pos-Zero)8/RConn1 -- VI sensor (Three-Phase)9/LConn1
  Bergeron Line (Pos-Zero)3/RConn1 -- VI sensor (Three-Phase)4/LConn1
  Bergeron Line (Pos-Zero)4/LConn1 -- VI sensor (Three-Phase)4/RConn1
  VI sensor (Three-Phase)3/LConn1 -- Bergeron Line (Pos-Zero)2/RConn1
  Bergeron Line (Pos-Zero)3/LConn1 -- VI sensor (Three-Phase)3/RConn1
  VI sensor (Three-Phase)2/LConn1 -- Bergeron Line (Pos-Zero)1/RConn1
  Bergeron Line (Pos-Zero)2/LConn1 -- VI sensor (Three-Phase)2/RConn1
  Bergeron Line (Pos-Zero)1/LConn1 -- VI sensor (Three-Phase)1/RConn1
  ~2/RConn1 -- Bergeron Line (Pos-Zero)9/RConn1
  VI sensor (Three-Phase)1/LConn1 -- Bergeron Line (Pos-Zero)10/RConn1
  VI sensor (Three-Phase)/LConn1 -- ~1/RConn1
  Bergeron Line (Pos-Zero)10/LConn1 -- VI sensor (Three-Phase)/RConn1

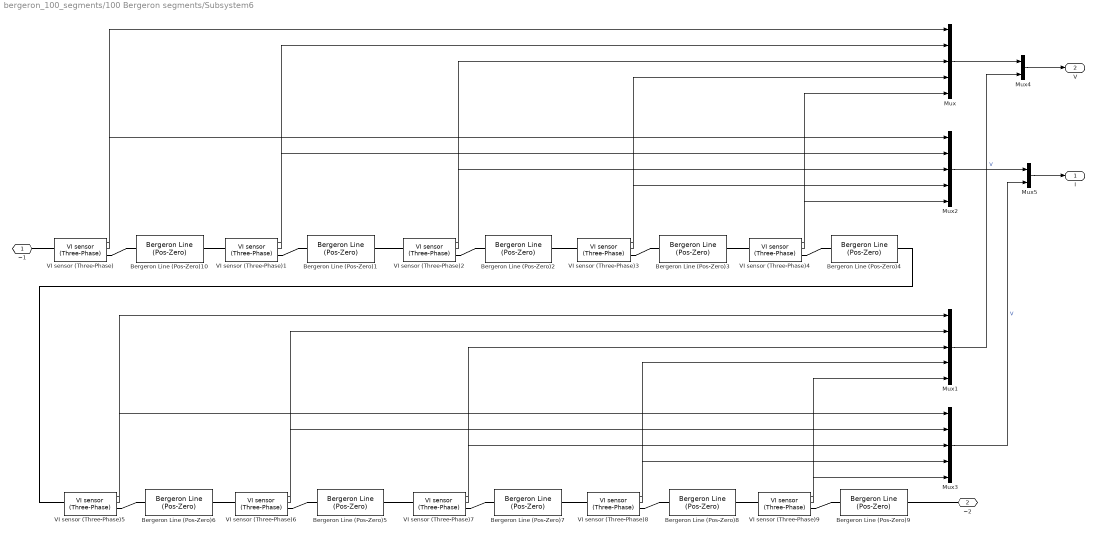
== system bergeron_100_segments/100 Bergeron segments/Subsystem6 ==
  Bergeron Line (Pos-Zero){1..10} (10 alike) : ee_lib_for_power_systems/Network Components/Bergeron Line (Pos-Zero)  length=length  R1_L1_C1=[R1 L1 C1]  R0_L0_C0=[R0 L0 C0]  Ts=Ts
      settings: SourceProductName=Support Library for Power Systems
  Mux{,1..3} (4 alike) : Mux  Inputs=5
  Mux4 : Mux  Inputs=2
  Mux5 : Mux  Inputs=2
  VI sensor (Three-Phase){,1..9} (10 alike) : ee_lib_for_power_systems/Sense and Measure/VI sensor (Three-Phase)  volt_meas=Phase-to-Ground (Phase Voltage)  meas_units=SI  Vnom=24e3  Pnom=100e6
      settings: SourceProductName=Support Library for Power Systems
  ~1 : PMIOPort  Side=Left
  ~2 : PMIOPort  Port=2  Side=Right
  I : Outport
  V : Outport  Port=2
  wires:
  VI sensor (Three-Phase)/1 -> Mux/1
  VI sensor (Three-Phase)1/1 -> Mux/2
  VI sensor (Three-Phase)2/1 -> Mux/3
  VI sensor (Three-Phase)3/1 -> Mux/4
  VI sensor (Three-Phase)4/1 -> Mux/5
  VI sensor (Three-Phase)/2 -> Mux2/1
  VI sensor (Three-Phase)1/2 -> Mux2/2
  VI sensor (Three-Phase)2/2 -> Mux2/3
  VI sensor (Three-Phase)3/2 -> Mux2/4
  VI sensor (Three-Phase)4/2 -> Mux2/5
  VI sensor (Three-Phase)5/1 -> Mux1/1
  VI sensor (Three-Phase)6/1 -> Mux1/2
  VI sensor (Three-Phase)7/1 -> Mux1/3
  VI sensor (Three-Phase)8/1 -> Mux1/4
  VI sensor (Three-Phase)9/1 -> Mux1/5
  VI sensor (Three-Phase)5/2 -> Mux3/1
  VI sensor (Three-Phase)6/2 -> Mux3/2
  VI sensor (Three-Phase)7/2 -> Mux3/3
  VI sensor (Three-Phase)8/2 -> Mux3/4
  VI sensor (Three-Phase)9/2 -> Mux3/5
  Mux/1 -> Mux4/1
  Mux1/1 -> Mux4/2
  Mux4/1 -> V/1
  Mux2/1 -> Mux5/1  "V"
  Mux3/1 -> Mux5/2  "V"
  Mux5/1 -> I/1
  connections:
  Bergeron Line (Pos-Zero)10/LConn1 -- VI sensor (Three-Phase)/RConn1
  VI sensor (Three-Phase)/LConn1 -- ~1/RConn1
  VI sensor (Three-Phase)1/LConn1 -- Bergeron Line (Pos-Zero)10/RConn1
  ~2/RConn1 -- Bergeron Line (Pos-Zero)9/RConn1
  Bergeron Line (Pos-Zero)1/LConn1 -- VI sensor (Three-Phase)1/RConn1
  Bergeron Line (Pos-Zero)2/LConn1 -- VI sensor (Three-Phase)2/RConn1
  VI sensor (Three-Phase)2/LConn1 -- Bergeron Line (Pos-Zero)1/RConn1
  Bergeron Line (Pos-Zero)3/LConn1 -- VI sensor (Three-Phase)3/RConn1
  VI sensor (Three-Phase)3/LConn1 -- Bergeron Line (Pos-Zero)2/RConn1
  Bergeron Line (Pos-Zero)4/LConn1 -- VI sensor (Three-Phase)4/RConn1
  Bergeron Line (Pos-Zero)3/RConn1 -- VI sensor (Three-Phase)4/LConn1
  Bergeron Line (Pos-Zero)8/RConn1 -- VI sensor (Three-Phase)9/LConn1
  Bergeron Line (Pos-Zero)9/LConn1 -- VI sensor (Three-Phase)9/RConn1
  VI sensor (Three-Phase)7/LConn1 -- Bergeron Line (Pos-Zero)5/RConn1
  Bergeron Line (Pos-Zero)8/LConn1 -- VI sensor (Three-Phase)8/RConn1
  Bergeron Line (Pos-Zero)7/LConn1 -- VI sensor (Three-Phase)7/RConn1
  Bergeron Line (Pos-Zero)5/LConn1 -- VI sensor (Three-Phase)6/RConn1
  VI sensor (Three-Phase)6/LConn1 -- Bergeron Line (Pos-Zero)6/RConn1
  Bergeron Line (Pos-Zero)6/LConn1 -- VI sensor (Three-Phase)5/RConn1
  VI sensor (Three-Phase)8/LConn1 -- Bergeron Line (Pos-Zero)7/RConn1
  VI sensor (Three-Phase)5/LConn1 -- Bergeron Line (Pos-Zero)4/RConn1

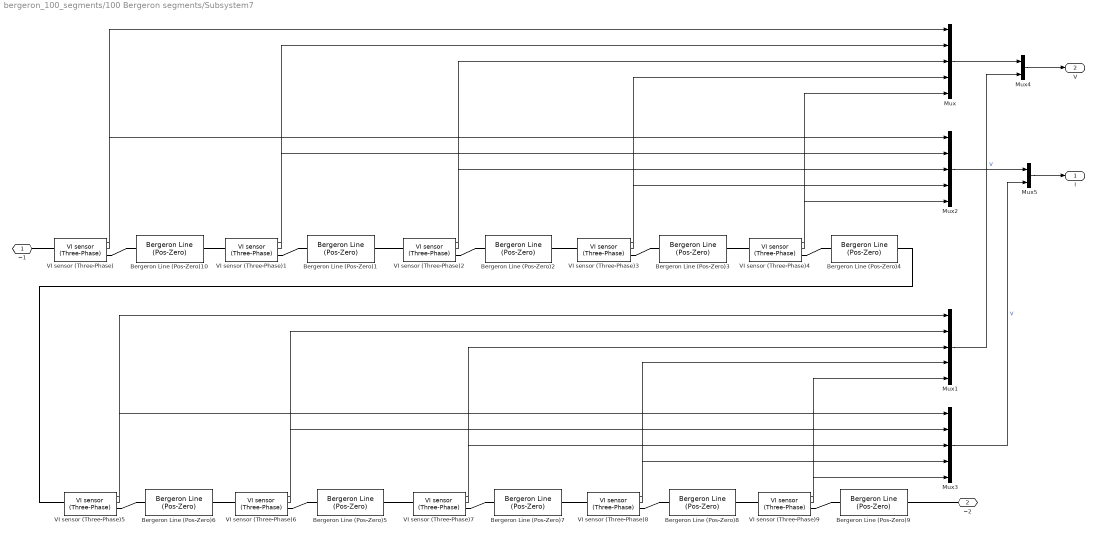
== system bergeron_100_segments/100 Bergeron segments/Subsystem7 ==
  Bergeron Line (Pos-Zero){1..10} (10 alike) : ee_lib_for_power_systems/Network Components/Bergeron Line (Pos-Zero)  length=length  R1_L1_C1=[R1 L1 C1]  R0_L0_C0=[R0 L0 C0]  Ts=Ts
      settings: SourceProductName=Support Library for Power Systems
  Mux{,1..3} (4 alike) : Mux  Inputs=5
  Mux4 : Mux  Inputs=2
  Mux5 : Mux  Inputs=2
  VI sensor (Three-Phase){,1..9} (10 alike) : ee_lib_for_power_systems/Sense and Measure/VI sensor (Three-Phase)  volt_meas=Phase-to-Ground (Phase Voltage)  meas_units=SI  Vnom=24e3  Pnom=100e6
      settings: SourceProductName=Support Library for Power Systems
  ~1 : PMIOPort  Side=Left
  ~2 : PMIOPort  Port=2  Side=Right
  I : Outport
  V : Outport  Port=2
  wires:
  Mux5/1 -> I/1
  Mux3/1 -> Mux5/2  "V"
  Mux2/1 -> Mux5/1  "V"
  Mux4/1 -> V/1
  Mux1/1 -> Mux4/2
  Mux/1 -> Mux4/1
  VI sensor (Three-Phase)9/2 -> Mux3/5
  VI sensor (Three-Phase)8/2 -> Mux3/4
  VI sensor (Three-Phase)7/2 -> Mux3/3
  VI sensor (Three-Phase)6/2 -> Mux3/2
  VI sensor (Three-Phase)5/2 -> Mux3/1
  VI sensor (Three-Phase)9/1 -> Mux1/5
  VI sensor (Three-Phase)8/1 -> Mux1/4
  VI sensor (Three-Phase)7/1 -> Mux1/3
  VI sensor (Three-Phase)6/1 -> Mux1/2
  VI sensor (Three-Phase)5/1 -> Mux1/1
  VI sensor (Three-Phase)4/2 -> Mux2/5
  VI sensor (Three-Phase)3/2 -> Mux2/4
  VI sensor (Three-Phase)2/2 -> Mux2/3
  VI sensor (Three-Phase)1/2 -> Mux2/2
  VI sensor (Three-Phase)/2 -> Mux2/1
  VI sensor (Three-Phase)4/1 -> Mux/5
  VI sensor (Three-Phase)3/1 -> Mux/4
  VI sensor (Three-Phase)2/1 -> Mux/3
  VI sensor (Three-Phase)1/1 -> Mux/2
  VI sensor (Three-Phase)/1 -> Mux/1
  connections:
  VI sensor (Three-Phase)5/LConn1 -- Bergeron Line (Pos-Zero)4/RConn1
  VI sensor (Three-Phase)8/LConn1 -- Bergeron Line (Pos-Zero)7/RConn1
  Bergeron Line (Pos-Zero)6/LConn1 -- VI sensor (Three-Phase)5/RConn1
  VI sensor (Three-Phase)6/LConn1 -- Bergeron Line (Pos-Zero)6/RConn1
  Bergeron Line (Pos-Zero)5/LConn1 -- VI sensor (Three-Phase)6/RConn1
  Bergeron Line (Pos-Zero)7/LConn1 -- VI sensor (Three-Phase)7/RConn1
  Bergeron Line (Pos-Zero)8/LConn1 -- VI sensor (Three-Phase)8/RConn1
  VI sensor (Three-Phase)7/LConn1 -- Bergeron Line (Pos-Zero)5/RConn1
  Bergeron Line (Pos-Zero)9/LConn1 -- VI sensor (Three-Phase)9/RConn1
  Bergeron Line (Pos-Zero)8/RConn1 -- VI sensor (Three-Phase)9/LConn1
  Bergeron Line (Pos-Zero)3/RConn1 -- VI sensor (Three-Phase)4/LConn1
  Bergeron Line (Pos-Zero)4/LConn1 -- VI sensor (Three-Phase)4/RConn1
  VI sensor (Three-Phase)3/LConn1 -- Bergeron Line (Pos-Zero)2/RConn1
  Bergeron Line (Pos-Zero)3/LConn1 -- VI sensor (Three-Phase)3/RConn1
  VI sensor (Three-Phase)2/LConn1 -- Bergeron Line (Pos-Zero)1/RConn1
  Bergeron Line (Pos-Zero)2/LConn1 -- VI sensor (Three-Phase)2/RConn1
  Bergeron Line (Pos-Zero)1/LConn1 -- VI sensor (Three-Phase)1/RConn1
  ~2/RConn1 -- Bergeron Line (Pos-Zero)9/RConn1
  VI sensor (Three-Phase)1/LConn1 -- Bergeron Line (Pos-Zero)10/RConn1
  VI sensor (Three-Phase)/LConn1 -- ~1/RConn1
  Bergeron Line (Pos-Zero)10/LConn1 -- VI sensor (Three-Phase)/RConn1

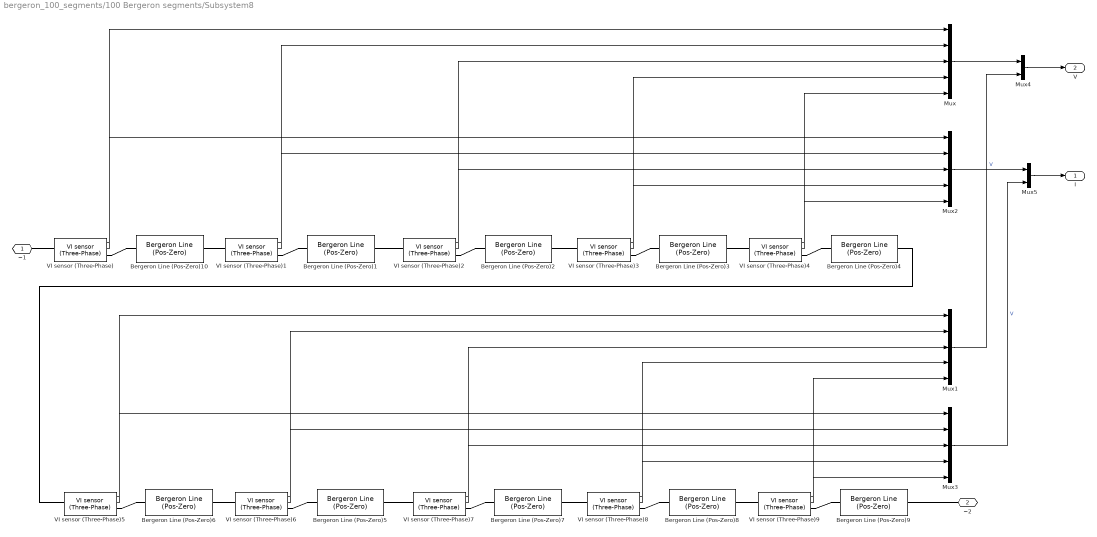
== system bergeron_100_segments/100 Bergeron segments/Subsystem8 ==
  Bergeron Line (Pos-Zero){1..10} (10 alike) : ee_lib_for_power_systems/Network Components/Bergeron Line (Pos-Zero)  length=length  R1_L1_C1=[R1 L1 C1]  R0_L0_C0=[R0 L0 C0]  Ts=Ts
      settings: SourceProductName=Support Library for Power Systems
  Mux{,1..3} (4 alike) : Mux  Inputs=5
  Mux4 : Mux  Inputs=2
  Mux5 : Mux  Inputs=2
  VI sensor (Three-Phase){,1..9} (10 alike) : ee_lib_for_power_systems/Sense and Measure/VI sensor (Three-Phase)  volt_meas=Phase-to-Ground (Phase Voltage)  meas_units=SI  Vnom=24e3  Pnom=100e6
      settings: SourceProductName=Support Library for Power Systems
  ~1 : PMIOPort  Side=Left
  ~2 : PMIOPort  Port=2  Side=Right
  I : Outport
  V : Outport  Port=2
  wires:
  VI sensor (Three-Phase)/1 -> Mux/1
  VI sensor (Three-Phase)1/1 -> Mux/2
  VI sensor (Three-Phase)2/1 -> Mux/3
  VI sensor (Three-Phase)3/1 -> Mux/4
  VI sensor (Three-Phase)4/1 -> Mux/5
  VI sensor (Three-Phase)/2 -> Mux2/1
  VI sensor (Three-Phase)1/2 -> Mux2/2
  VI sensor (Three-Phase)2/2 -> Mux2/3
  VI sensor (Three-Phase)3/2 -> Mux2/4
  VI sensor (Three-Phase)4/2 -> Mux2/5
  VI sensor (Three-Phase)5/1 -> Mux1/1
  VI sensor (Three-Phase)6/1 -> Mux1/2
  VI sensor (Three-Phase)7/1 -> Mux1/3
  VI sensor (Three-Phase)8/1 -> Mux1/4
  VI sensor (Three-Phase)9/1 -> Mux1/5
  VI sensor (Three-Phase)5/2 -> Mux3/1
  VI sensor (Three-Phase)6/2 -> Mux3/2
  VI sensor (Three-Phase)7/2 -> Mux3/3
  VI sensor (Three-Phase)8/2 -> Mux3/4
  VI sensor (Three-Phase)9/2 -> Mux3/5
  Mux/1 -> Mux4/1
  Mux1/1 -> Mux4/2
  Mux4/1 -> V/1
  Mux2/1 -> Mux5/1  "V"
  Mux3/1 -> Mux5/2  "V"
  Mux5/1 -> I/1
  connections:
  Bergeron Line (Pos-Zero)10/LConn1 -- VI sensor (Three-Phase)/RConn1
  VI sensor (Three-Phase)/LConn1 -- ~1/RConn1
  VI sensor (Three-Phase)1/LConn1 -- Bergeron Line (Pos-Zero)10/RConn1
  ~2/RConn1 -- Bergeron Line (Pos-Zero)9/RConn1
  Bergeron Line (Pos-Zero)1/LConn1 -- VI sensor (Three-Phase)1/RConn1
  Bergeron Line (Pos-Zero)2/LConn1 -- VI sensor (Three-Phase)2/RConn1
  VI sensor (Three-Phase)2/LConn1 -- Bergeron Line (Pos-Zero)1/RConn1
  Bergeron Line (Pos-Zero)3/LConn1 -- VI sensor (Three-Phase)3/RConn1
  VI sensor (Three-Phase)3/LConn1 -- Bergeron Line (Pos-Zero)2/RConn1
  Bergeron Line (Pos-Zero)4/LConn1 -- VI sensor (Three-Phase)4/RConn1
  Bergeron Line (Pos-Zero)3/RConn1 -- VI sensor (Three-Phase)4/LConn1
  Bergeron Line (Pos-Zero)8/RConn1 -- VI sensor (Three-Phase)9/LConn1
  Bergeron Line (Pos-Zero)9/LConn1 -- VI sensor (Three-Phase)9/RConn1
  VI sensor (Three-Phase)7/LConn1 -- Bergeron Line (Pos-Zero)5/RConn1
  Bergeron Line (Pos-Zero)8/LConn1 -- VI sensor (Three-Phase)8/RConn1
  Bergeron Line (Pos-Zero)7/LConn1 -- VI sensor (Three-Phase)7/RConn1
  Bergeron Line (Pos-Zero)5/LConn1 -- VI sensor (Three-Phase)6/RConn1
  VI sensor (Three-Phase)6/LConn1 -- Bergeron Line (Pos-Zero)6/RConn1
  Bergeron Line (Pos-Zero)6/LConn1 -- VI sensor (Three-Phase)5/RConn1
  VI sensor (Three-Phase)8/LConn1 -- Bergeron Line (Pos-Zero)7/RConn1
  VI sensor (Three-Phase)5/LConn1 -- Bergeron Line (Pos-Zero)4/RConn1

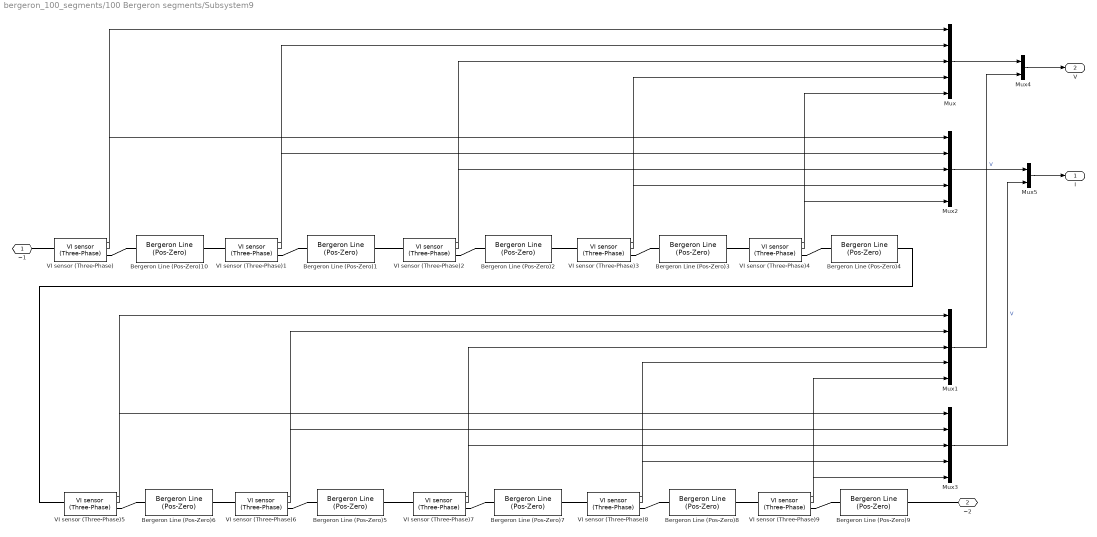
== system bergeron_100_segments/100 Bergeron segments/Subsystem9 ==
  Bergeron Line (Pos-Zero){1..10} (10 alike) : ee_lib_for_power_systems/Network Components/Bergeron Line (Pos-Zero)  length=length  R1_L1_C1=[R1 L1 C1]  R0_L0_C0=[R0 L0 C0]  Ts=Ts
      settings: SourceProductName=Support Library for Power Systems
  Mux{,1..3} (4 alike) : Mux  Inputs=5
  Mux4 : Mux  Inputs=2
  Mux5 : Mux  Inputs=2
  VI sensor (Three-Phase){,1..9} (10 alike) : ee_lib_for_power_systems/Sense and Measure/VI sensor (Three-Phase)  volt_meas=Phase-to-Ground (Phase Voltage)  meas_units=SI  Vnom=24e3  Pnom=100e6
      settings: SourceProductName=Support Library for Power Systems
  ~1 : PMIOPort  Side=Left
  ~2 : PMIOPort  Port=2  Side=Right
  I : Outport
  V : Outport  Port=2
  wires:
  Mux5/1 -> I/1
  Mux3/1 -> Mux5/2  "V"
  Mux2/1 -> Mux5/1  "V"
  Mux4/1 -> V/1
  Mux1/1 -> Mux4/2
  Mux/1 -> Mux4/1
  VI sensor (Three-Phase)9/2 -> Mux3/5
  VI sensor (Three-Phase)8/2 -> Mux3/4
  VI sensor (Three-Phase)7/2 -> Mux3/3
  VI sensor (Three-Phase)6/2 -> Mux3/2
  VI sensor (Three-Phase)5/2 -> Mux3/1
  VI sensor (Three-Phase)9/1 -> Mux1/5
  VI sensor (Three-Phase)8/1 -> Mux1/4
  VI sensor (Three-Phase)7/1 -> Mux1/3
  VI sensor (Three-Phase)6/1 -> Mux1/2
  VI sensor (Three-Phase)5/1 -> Mux1/1
  VI sensor (Three-Phase)4/2 -> Mux2/5
  VI sensor (Three-Phase)3/2 -> Mux2/4
  VI sensor (Three-Phase)2/2 -> Mux2/3
  VI sensor (Three-Phase)1/2 -> Mux2/2
  VI sensor (Three-Phase)/2 -> Mux2/1
  VI sensor (Three-Phase)4/1 -> Mux/5
  VI sensor (Three-Phase)3/1 -> Mux/4
  VI sensor (Three-Phase)2/1 -> Mux/3
  VI sensor (Three-Phase)1/1 -> Mux/2
  VI sensor (Three-Phase)/1 -> Mux/1
  connections:
  VI sensor (Three-Phase)5/LConn1 -- Bergeron Line (Pos-Zero)4/RConn1
  VI sensor (Three-Phase)8/LConn1 -- Bergeron Line (Pos-Zero)7/RConn1
  Bergeron Line (Pos-Zero)6/LConn1 -- VI sensor (Three-Phase)5/RConn1
  VI sensor (Three-Phase)6/LConn1 -- Bergeron Line (Pos-Zero)6/RConn1
  Bergeron Line (Pos-Zero)5/LConn1 -- VI sensor (Three-Phase)6/RConn1
  Bergeron Line (Pos-Zero)7/LConn1 -- VI sensor (Three-Phase)7/RConn1
  Bergeron Line (Pos-Zero)8/LConn1 -- VI sensor (Three-Phase)8/RConn1
  VI sensor (Three-Phase)7/LConn1 -- Bergeron Line (Pos-Zero)5/RConn1
  Bergeron Line (Pos-Zero)9/LConn1 -- VI sensor (Three-Phase)9/RConn1
  Bergeron Line (Pos-Zero)8/RConn1 -- VI sensor (Three-Phase)9/LConn1
  Bergeron Line (Pos-Zero)3/RConn1 -- VI sensor (Three-Phase)4/LConn1
  Bergeron Line (Pos-Zero)4/LConn1 -- VI sensor (Three-Phase)4/RConn1
  VI sensor (Three-Phase)3/LConn1 -- Bergeron Line (Pos-Zero)2/RConn1
  Bergeron Line (Pos-Zero)3/LConn1 -- VI sensor (Three-Phase)3/RConn1
  VI sensor (Three-Phase)2/LConn1 -- Bergeron Line (Pos-Zero)1/RConn1
  Bergeron Line (Pos-Zero)2/LConn1 -- VI sensor (Three-Phase)2/RConn1
  Bergeron Line (Pos-Zero)1/LConn1 -- VI sensor (Three-Phase)1/RConn1
  ~2/RConn1 -- Bergeron Line (Pos-Zero)9/RConn1
  VI sensor (Three-Phase)1/LConn1 -- Bergeron Line (Pos-Zero)10/RConn1
  VI sensor (Three-Phase)/LConn1 -- ~1/RConn1
  Bergeron Line (Pos-Zero)10/LConn1 -- VI sensor (Three-Phase)/RConn1
